simulink model "Copy_of_AB_Final_of_MPC_Bandwidth_Result"  (R2022b)
settings: Solver=FixedStepDiscrete  StartTime=0.0  StopTime=Inf  FixedStep=100e-6  RelTol=1e-3  EnableMultiTasking=on
undefined symbols (not defined in the file): C28x, CPU1, CPU2, CurrentBypassValue, DiscIntNeverNeededParam, Down, GPTRIP1SEL, TZ1, Up
libraries: c2802xlib x31, simulink x22, dspstat3 x17, dspsigops x9, c2837xDlib x6, c280xlib x5, PID_Lib x2, c2000lib x1, spsAlphaBetaZerotoabcLib x1, spsAlphaBetaZerotodq0Lib x1
(part 3 of 8)

== system Copy_of_AB_Final_of_MPC_Bandwidth_Result/Subsystem1/Subsystem ==
  PWM1 : Inport
  PWM2 : Inport  Port=2
  PWM3 : Inport  Port=3
  Trip : Inport  Port=4
  Constant12 : Constant  Value=uint32(4999)
  Constant13 : Constant  Value=uint32(0)
  Constant16 : Constant  Value=uint32(4999)
  Constant17 : Constant  Value=uint32(0)
  Constant6 : Constant  Value=uint32(4999)
  Constant7 : Constant  Value=uint32(0)
  Data Type Conversion18 : DataTypeConversion  OutDataTypeStr=uint32  SaturateOnIntegerOverflow=off  RndMeth=Floor
  Data Type Conversion19 : DataTypeConversion  OutDataTypeStr=uint32  SaturateOnIntegerOverflow=off  RndMeth=Floor
  Data Type Conversion5 : DataTypeConversion  OutDataTypeStr=uint32  SaturateOnIntegerOverflow=off  RndMeth=Floor
  From : From
  From1 : From
  From2 : From
  Gain : Gain
  Goto : Goto
  Saturation Dynamic1 : simulink/Discontinuities/Saturation Dynamic  OutMin=[]  OutMax=[]  OutDataTypeStr=Inherit: Same as second input  OutDataType=fixdt(1, 16)  OutScaling=2^-10  DoSatur=off
  Saturation Dynamic2 : simulink/Discontinuities/Saturation Dynamic  OutMin=[]  OutMax=[]  OutDataTypeStr=Inherit: Same as second input  OutDataType=fixdt(1, 16)  OutScaling=2^-10  DoSatur=off
  Saturation Dynamic3 : simulink/Discontinuities/Saturation Dynamic  OutMin=[]  OutMax=[]  OutDataTypeStr=Inherit: Same as second input  OutDataType=fixdt(1, 16)  OutScaling=2^-10  DoSatur=off
  ePWM5 : c2802xlib/ePWM  PwmType=C2000_Type4  useModule=ePWM1  ePWMxLINKTBPRD=Not Linked  periodUnits=Clock cycles  timerSource=Specify via dialog  timerPeriod_clk=5000  timerPeriod_sec=0.0001  tbshadow=Counter equals to zero  countingMode=Up-Down  phaseActiveEnable=Disable  phaseDirection=Count down after sync  phaseActive=0  synchronizationEnable=off  dcaevt1Sync=off  dcbevt1Sync=off  synchronizationOption=Disable  dcbevt1SyncOut=off  dcaevt1SyncOut=off  cmpdSyncOut=off  cmpcSyncOut=off  cmpbSyncOut=off  zeroSyncOut=off  swfSyncOut=off  perSynchronizationOption=Counter equals to period (CTR=PRD)  clockPrescale=1  HSclockPrescale=1  enswap=off  ePWMxAStatus=on  ePWMxAactionLogic1=Do nothing  ePWMxAactionLogic2=Do nothing  ePWMxAactionLogic3=Clear  ePWMxAactionLogic4=Set  ePWMxAactionLogic5=Do nothing  ePWMxAactionLogic6=Do nothing  ePWMxACSFenable=off  ePWMxACSFvalue=Forcing disable  ePWMxASFreload=Zero  ePWMxBStatus=off  ePWMxBactionLogic1=Set  ePWMxBactionLogic2=Clear  ePWMxBactionLogic3=Do nothing  ePWMxBactionLogic4=Do nothing  ePWMxBactionLogic5=Clear  ePWMxBactionLogic6=Set  ePWMxBCSFenable=off  ePWMxBCSFvalue=Forcing disable  ePWMxBSFreload=Zero  ePWNxBOutWay=off  ePWMxLINKCMPA=Not Linked  CMPAUnits=Clock cycles  CMPASource=Input port  CMPAValue_per=50  CMPAValue_clk=0  enCMPAshadow=Counter equals to zero (CTR=Zero)  ePWMxLINKCMPB=Not Linked  CMPBUnits=Clock cycles  CMPBSource=Specify via dialog  CMPBValue_per=50  CMPBValue_clk=0  enCMPBshadow=Counter equals to zero (CTR=Zero)  ePWMxLINKCMPC=Not Linked  CMPCUnits=Clock cycles  CMPCSource=Specify via dialog  CMPCValue_per=50  CMPCValue_clk=0  enCMPCshadow=Counter equals to zero (CTR=Zero)  ePWMxLINKCMPD=Not Linked  CMPDUnits=Clock cycles  CMPDSource=Specify via dialog  CMPDValue_per=50  CMPDValue_clk=32000  enCMPDshadow=Counter equals to zero (CTR=Zero)  enableDBePWMxA=on  enableDBePWMxB=on  enhalfcycle=off  DBpolarity=Active high complementary (AHC)  DBedgeDelay=Positive  DBSource_ePWMxA=ePWMxA  DBSource_ePWMxB=ePWMxA  DBPeriodUnits=Seconds  DBperiodSource=Specify via dialog  REDperiod=250  FEDperiod=250  REDperiod_sec=500e-9  FEDperiod_sec=500e-9  LoadModeDBRED=Immediate without using shadow  LoadModeDBFED=Immediate without using shadow  adcstartModuleA=on  adcrequestEventA=First event  adcstartEventA=Digital Compare Module A Event 1 start of conversion (DCAEVT1.soc)  adcstartEventA_type2=Counter equals to period (CTR=PRD)  adcstartModuleB=off  adcrequestEventB=First event  adcstartEventB=Counter equals to zero (CTR=Zero)  adcstartEventB_type2=Counter equals to zero (CTR=Zero)  intEn=off  intPrd=First event  intSel=Counter equals to zero (CTR=Zero)  intSel_type2=Counter equals to zero (CTR=Zero)  hrpe=off  enHRPWM=off  HRPWM_LoadMode=Counter equals to period (CTR=PRD)  HRPWM_CTLMode=Duty or Period control mode  HRPWM_EDGMode=Both edge  hrpeb=off  enHRPWMB=off  HRPWM_LoadModeB=Counter equals to zero (CTR=ZERO)  HRPWM_CTLModeB=Duty or Period control mode  HRPWM_EDGModeB=Both edge  enHRDBRED=off  enHRDBFED=off  enSFO=on  enautoconv=on  chopperEnable=off  chopperFrequency=1  chopperFirstwidth=1  chopperDuty=12.5%  tripZonesource=Input port  tzselOSHT1=off  tzselOSHT2=off  tzselOSHT3=off  tzselOSHDCAEV1=off  tzselOSHDCBEV1=off  tzselCBC1=off  tzselCBC2=off  tzselCBC3=off  tzselCBCDCAEV2=off  tzselCBCDCBEV2=off  tzselOSHT4=off  tzselOSHT5=off  tzselOSHT6=off  tzselCBC4=off  tzselCBC5=off  tzselCBC6=off  enTzOstIntr=off  enTzCbcIntr=off  enTzDCAEVT1Intr=off  enTzDCAEVT2Intr=off  enTzDCBEVT1Intr=off  enTzDCBEVT2Intr=off  ePWMxAforced=Low  ePWMxBforced=Low  DCAEVT1forced=No action  DCBEVT1forced=No action  DCAEVT2forced=No action  DCBEVT2forced=No action  dcah=Trip Zone 1 input (TZ1)  dcal=Trip Zone 2 input (TZ2)  dcbh=Trip Zone 1 input (TZ1)  dcbl=Trip Zone 2 input (TZ2)  dcah_type2=GPTRIP1SEL/(TZ1)  dcal_type2=GPTRIP1SEL/(TZ1)  dcbh_type2=GPTRIP1SEL/(TZ1)  dcbl_type2=GPTRIP1SEL/(TZ1)  gendcaevt1=Event disabled  gendcaevt2=Event disabled  gendcbevt1=Event disabled  gendcbevt2=Event disabled  dcaevt1src=DCAEVT1 with sync  dcaevt2src=DCAEVT2 with sync  dcbevt1src=DCBEVT1 with sync  dcbevt2src=DCBEVT2 with sync  pulsesel=Counter equals to zero (CTR=Zero)  blankinv=off  blankoffset=0  blankwidth=0  evsrcsel=Filtered version of DCAEVT1 (DCAEVT1FILT)  encape=off
  ePWM6 : c2802xlib/ePWM  PwmType=C2000_Type4  useModule=ePWM2  ePWMxLINKTBPRD=Not Linked  periodUnits=Clock cycles  timerSource=Specify via dialog  timerPeriod_clk=5000  timerPeriod_sec=0.0001  tbshadow=Counter equals to zero  countingMode=Up-Down  phaseActiveEnable=Disable  phaseDirection=Count down after sync  phaseActive=0  synchronizationEnable=off  dcaevt1Sync=off  dcbevt1Sync=off  synchronizationOption=Disable  dcbevt1SyncOut=off  dcaevt1SyncOut=off  cmpdSyncOut=off  cmpcSyncOut=off  cmpbSyncOut=off  zeroSyncOut=off  swfSyncOut=off  perSynchronizationOption=Counter equals to period (CTR=PRD)  clockPrescale=1  HSclockPrescale=1  enswap=off  ePWMxAStatus=on  ePWMxAactionLogic1=Do nothing  ePWMxAactionLogic2=Do nothing  ePWMxAactionLogic3=Clear  ePWMxAactionLogic4=Set  ePWMxAactionLogic5=Do nothing  ePWMxAactionLogic6=Do nothing  ePWMxACSFenable=off  ePWMxACSFvalue=Forcing disable  ePWMxASFreload=Zero  ePWMxBStatus=off  ePWMxBactionLogic1=Set  ePWMxBactionLogic2=Clear  ePWMxBactionLogic3=Do nothing  ePWMxBactionLogic4=Do nothing  ePWMxBactionLogic5=Clear  ePWMxBactionLogic6=Set  ePWMxBCSFenable=off  ePWMxBCSFvalue=Forcing disable  ePWMxBSFreload=Zero  ePWNxBOutWay=off  ePWMxLINKCMPA=Not Linked  CMPAUnits=Clock cycles  CMPASource=Input port  CMPAValue_per=50  CMPAValue_clk=0  enCMPAshadow=Counter equals to zero (CTR=Zero)  ePWMxLINKCMPB=Not Linked  CMPBUnits=Clock cycles  CMPBSource=Specify via dialog  CMPBValue_per=50  CMPBValue_clk=0  enCMPBshadow=Counter equals to zero (CTR=Zero)  ePWMxLINKCMPC=Not Linked  CMPCUnits=Clock cycles  CMPCSource=Specify via dialog  CMPCValue_per=50  CMPCValue_clk=0  enCMPCshadow=Counter equals to zero (CTR=Zero)  ePWMxLINKCMPD=Not Linked  CMPDUnits=Clock cycles  CMPDSource=Specify via dialog  CMPDValue_per=50  CMPDValue_clk=32000  enCMPDshadow=Counter equals to zero (CTR=Zero)  enableDBePWMxA=on  enableDBePWMxB=on  enhalfcycle=off  DBpolarity=Active high complementary (AHC)  DBedgeDelay=Positive  DBSource_ePWMxA=ePWMxA  DBSource_ePWMxB=ePWMxA  DBPeriodUnits=Seconds  DBperiodSource=Specify via dialog  REDperiod=250  FEDperiod=250  REDperiod_sec=500e-9  FEDperiod_sec=500e-9  LoadModeDBRED=Immediate without using shadow  LoadModeDBFED=Immediate without using shadow  adcstartModuleA=off  adcrequestEventA=First event  adcstartEventA=Digital Compare Module A Event 1 start of conversion (DCAEVT1.soc)  adcstartEventA_type2=Counter equals to zero (CTR=Zero)  adcstartModuleB=off  adcrequestEventB=First event  adcstartEventB=Counter equals to zero (CTR=Zero)  adcstartEventB_type2=Counter equals to zero (CTR=Zero)  intEn=off  intPrd=First event  intSel=Counter equals to zero (CTR=Zero)  intSel_type2=Counter equals to zero (CTR=Zero)  hrpe=off  enHRPWM=off  HRPWM_LoadMode=Counter equals to period (CTR=PRD)  HRPWM_CTLMode=Duty or Period control mode  HRPWM_EDGMode=Both edge  hrpeb=off  enHRPWMB=off  HRPWM_LoadModeB=Counter equals to zero (CTR=ZERO)  HRPWM_CTLModeB=Duty or Period control mode  HRPWM_EDGModeB=Both edge  enHRDBRED=off  enHRDBFED=off  enSFO=on  enautoconv=on  chopperEnable=off  chopperFrequency=1  chopperFirstwidth=1  chopperDuty=12.5%  tripZonesource=Input port  tzselOSHT1=off  tzselOSHT2=off  tzselOSHT3=off  tzselOSHDCAEV1=off  tzselOSHDCBEV1=off  tzselCBC1=off  tzselCBC2=off  tzselCBC3=off  tzselCBCDCAEV2=off  tzselCBCDCBEV2=off  tzselOSHT4=off  tzselOSHT5=off  tzselOSHT6=off  tzselCBC4=off  tzselCBC5=off  tzselCBC6=off  enTzOstIntr=off  enTzCbcIntr=off  enTzDCAEVT1Intr=off  enTzDCAEVT2Intr=off  enTzDCBEVT1Intr=off  enTzDCBEVT2Intr=off  ePWMxAforced=Low  ePWMxBforced=Low  DCAEVT1forced=No action  DCBEVT1forced=No action  DCAEVT2forced=No action  DCBEVT2forced=No action  dcah=Trip Zone 1 input (TZ1)  dcal=Trip Zone 2 input (TZ2)  dcbh=Trip Zone 1 input (TZ1)  dcbl=Trip Zone 2 input (TZ2)  dcah_type2=GPTRIP1SEL/(TZ1)  dcal_type2=GPTRIP1SEL/(TZ1)  dcbh_type2=GPTRIP1SEL/(TZ1)  dcbl_type2=GPTRIP1SEL/(TZ1)  gendcaevt1=Event disabled  gendcaevt2=Event disabled  gendcbevt1=Event disabled  gendcbevt2=Event disabled  dcaevt1src=DCAEVT1 with sync  dcaevt2src=DCAEVT2 with sync  dcbevt1src=DCBEVT1 with sync  dcbevt2src=DCBEVT2 with sync  pulsesel=Counter equals to zero (CTR=Zero)  blankinv=off  blankoffset=0  blankwidth=0  evsrcsel=Filtered version of DCAEVT1 (DCAEVT1FILT)  encape=off
  ePWM7 : c2802xlib/ePWM  PwmType=C2000_Type4  useModule=ePWM3  ePWMxLINKTBPRD=Not Linked  periodUnits=Clock cycles  timerSource=Specify via dialog  timerPeriod_clk=5000  timerPeriod_sec=0.0001  tbshadow=Counter equals to zero  countingMode=Up-Down  phaseActiveEnable=Disable  phaseDirection=Count down after sync  phaseActive=0  synchronizationEnable=off  dcaevt1Sync=off  dcbevt1Sync=off  synchronizationOption=Disable  dcbevt1SyncOut=off  dcaevt1SyncOut=off  cmpdSyncOut=off  cmpcSyncOut=off  cmpbSyncOut=off  zeroSyncOut=off  swfSyncOut=off  perSynchronizationOption=Counter equals to period (CTR=PRD)  clockPrescale=1  HSclockPrescale=1  enswap=off  ePWMxAStatus=on  ePWMxAactionLogic1=Do nothing  ePWMxAactionLogic2=Do nothing  ePWMxAactionLogic3=Clear  ePWMxAactionLogic4=Set  ePWMxAactionLogic5=Do nothing  ePWMxAactionLogic6=Do nothing  ePWMxACSFenable=off  ePWMxACSFvalue=Forcing disable  ePWMxASFreload=Zero  ePWMxBStatus=off  ePWMxBactionLogic1=Set  ePWMxBactionLogic2=Clear  ePWMxBactionLogic3=Do nothing  ePWMxBactionLogic4=Do nothing  ePWMxBactionLogic5=Clear  ePWMxBactionLogic6=Set  ePWMxBCSFenable=off  ePWMxBCSFvalue=Forcing disable  ePWMxBSFreload=Zero  ePWNxBOutWay=off  ePWMxLINKCMPA=Not Linked  CMPAUnits=Clock cycles  CMPASource=Input port  CMPAValue_per=50  CMPAValue_clk=0  enCMPAshadow=Counter equals to zero (CTR=Zero)  ePWMxLINKCMPB=Not Linked  CMPBUnits=Clock cycles  CMPBSource=Specify via dialog  CMPBValue_per=50  CMPBValue_clk=0  enCMPBshadow=Counter equals to zero (CTR=Zero)  ePWMxLINKCMPC=Not Linked  CMPCUnits=Clock cycles  CMPCSource=Specify via dialog  CMPCValue_per=50  CMPCValue_clk=0  enCMPCshadow=Counter equals to zero (CTR=Zero)  ePWMxLINKCMPD=Not Linked  CMPDUnits=Clock cycles  CMPDSource=Specify via dialog  CMPDValue_per=50  CMPDValue_clk=32000  enCMPDshadow=Counter equals to zero (CTR=Zero)  enableDBePWMxA=on  enableDBePWMxB=on  enhalfcycle=off  DBpolarity=Active high complementary (AHC)  DBedgeDelay=Positive  DBSource_ePWMxA=ePWMxA  DBSource_ePWMxB=ePWMxA  DBPeriodUnits=Seconds  DBperiodSource=Specify via dialog  REDperiod=250  FEDperiod=250  REDperiod_sec=500e-9  FEDperiod_sec=500e-9  LoadModeDBRED=Immediate without using shadow  LoadModeDBFED=Immediate without using shadow  adcstartModuleA=off  adcrequestEventA=First event  adcstartEventA=Digital Compare Module A Event 1 start of conversion (DCAEVT1.soc)  adcstartEventA_type2=Counter equals to zero (CTR=Zero)  adcstartModuleB=off  adcrequestEventB=First event  adcstartEventB=Counter equals to zero (CTR=Zero)  adcstartEventB_type2=Counter equals to zero (CTR=Zero)  intEn=off  intPrd=First event  intSel=Counter equals to zero (CTR=Zero)  intSel_type2=Counter equals to zero (CTR=Zero)  hrpe=off  enHRPWM=off  HRPWM_LoadMode=Counter equals to period (CTR=PRD)  HRPWM_CTLMode=Duty or Period control mode  HRPWM_EDGMode=Both edge  hrpeb=off  enHRPWMB=off  HRPWM_LoadModeB=Counter equals to zero (CTR=ZERO)  HRPWM_CTLModeB=Duty or Period control mode  HRPWM_EDGModeB=Both edge  enHRDBRED=off  enHRDBFED=off  enSFO=on  enautoconv=on  chopperEnable=off  chopperFrequency=1  chopperFirstwidth=1  chopperDuty=12.5%  tripZonesource=Input port  tzselOSHT1=off  tzselOSHT2=off  tzselOSHT3=off  tzselOSHDCAEV1=off  tzselOSHDCBEV1=off  tzselCBC1=off  tzselCBC2=off  tzselCBC3=off  tzselCBCDCAEV2=off  tzselCBCDCBEV2=off  tzselOSHT4=off  tzselOSHT5=off  tzselOSHT6=off  tzselCBC4=off  tzselCBC5=off  tzselCBC6=off  enTzOstIntr=off  enTzCbcIntr=off  enTzDCAEVT1Intr=off  enTzDCAEVT2Intr=off  enTzDCBEVT1Intr=off  enTzDCBEVT2Intr=off  ePWMxAforced=Low  ePWMxBforced=Low  DCAEVT1forced=No action  DCBEVT1forced=No action  DCAEVT2forced=No action  DCBEVT2forced=No action  dcah=Trip Zone 1 input (TZ1)  dcal=Trip Zone 2 input (TZ2)  dcbh=Trip Zone 1 input (TZ1)  dcbl=Trip Zone 2 input (TZ2)  dcah_type2=GPTRIP1SEL/(TZ1)  dcal_type2=GPTRIP1SEL/(TZ1)  dcbh_type2=GPTRIP1SEL/(TZ1)  dcbl_type2=GPTRIP1SEL/(TZ1)  gendcaevt1=Event disabled  gendcaevt2=Event disabled  gendcbevt1=Event disabled  gendcbevt2=Event disabled  dcaevt1src=DCAEVT1 with sync  dcaevt2src=DCAEVT2 with sync  dcbevt1src=DCBEVT1 with sync  dcbevt2src=DCBEVT2 with sync  pulsesel=Counter equals to zero (CTR=Zero)  blankinv=off  blankoffset=0  blankwidth=0  evsrcsel=Filtered version of DCAEVT1 (DCAEVT1FILT)  encape=off
  wires:
  Data Type Conversion5/1 -> ePWM5/1
  Constant13/1 -> Saturation Dynamic3/3
  Constant6/1 -> Saturation Dynamic1/1
  Constant12/1 -> Saturation Dynamic3/1
  Constant7/1 -> Saturation Dynamic1/3
  Saturation Dynamic1/1 -> Data Type Conversion5/1
  Constant16/1 -> Saturation Dynamic2/1
  Data Type Conversion18/1 -> ePWM6/1
  Data Type Conversion19/1 -> ePWM7/1
  Saturation Dynamic3/1 -> Data Type Conversion19/1
  Constant17/1 -> Saturation Dynamic2/3
  Saturation Dynamic2/1 -> Data Type Conversion18/1
  PWM1/1 -> Saturation Dynamic1/2
  PWM3/1 -> Saturation Dynamic3/2
  PWM2/1 -> Saturation Dynamic2/2
  From/1 -> ePWM5/2
  From1/1 -> ePWM6/2
  From2/1 -> ePWM7/2
  Trip/1 -> Gain/1
  Gain/1 -> Goto/1

== system Copy_of_AB_Final_of_MPC_Bandwidth_Result/Subsystem1/Subsystem1 ==
  In1 : Inport
  In2 : Inport  Port=2
  Enable : EnablePort  StatesWhenEnabling=reset
  Add : Sum
  Add3 : Sum
  Bus Creator : BusCreator  Inputs=2
  Bus Selector1 : BusSelector  OutputSignals=signal1,signal2
  CodeGeneration : Subsystem  TreatAsAtomicUnit=on
  Constant3 : Constant  Value=100  OutDataTypeStr=single
  Counter Limited : simulink/Sources/Counter Limited  uplimit=599  tsamp=-1
  Data : Subsystem  TreatAsAtomicUnit=on
  Data_Conditioning : Subsystem
  End : Subsystem  TreatAsAtomicUnit=on
  Gain6 : Gain  Gain=1000  OutDataTypeStr=single
  Gain7 : Gain  Gain=1000  OutDataTypeStr=single
  If : If  IfExpression=u1 == 0  ElseIfExpressions=u1 == 599
  Merge : Merge  Inputs=3
  Merge1 : Merge  Inputs=3
  Mux : Mux  Inputs=2
  Mux1 : Mux  Inputs=2
  Start : Subsystem  TreatAsAtomicUnit=on
  Width : Width  OutDataTypeMode=All ports same datatype  DataType=uint16
  wires:
  Start/2(Iteration) -> Merge1/1
  Constant3/1 -> Add/2, Add3/1
  Counter Limited/1 -> If/1
  Data_Conditioning/1(Out1) -> Width/1, Start/1(Data), End/1(Data), Data/1(Data)
  End/1(Data_out) -> Merge/2
  End/2(Iteration) -> Merge1/2
  If/3 -> Data/Action
  Add/1 -> Gain6/1
  Data/2(Iteration) -> Merge1/3
  Merge1/1 -> Mux/2  "SCI_Tx_Iteration"
  Bus Selector1/1 -> Add/1  "<signal1>"
  Start/1(Data_out) -> Merge/1
  Add3/1 -> Gain7/1
  Mux1/1 -> Data_Conditioning/1(In1)
  In1/1 -> Bus Creator/1
  Merge/1 -> Mux/1  "SCI_Tx_Data"
  If/2 -> End/Action
  Data/1(Data_out) -> Merge/3
  Bus Creator/1 -> Bus Selector1/1
  Width/1 -> Start/2(Data_width), Data/2(Data_width), End/2(Data_width)
  Mux/1 -> CodeGeneration/1(Input)
  In2/1 -> Bus Creator/2
  Gain7/1 -> Mux1/2
  Bus Selector1/2 -> Add3/2  "<signal2>"
  If/1 -> Start/Action
  Gain6/1 -> Mux1/1

== system Copy_of_AB_Final_of_MPC_Bandwidth_Result/Subsystem1/Subsystem2 ==
  In1 : Inport
  In2 : Inport  Port=2
  Enable : EnablePort  StatesWhenEnabling=reset
  Add : Sum
  Add3 : Sum
  Bus Creator : BusCreator  Inputs=2
  Bus Selector1 : BusSelector  OutputSignals=signal1,signal2
  CodeGeneration : Subsystem  TreatAsAtomicUnit=on
  Constant3 : Constant  Value=10  OutDataTypeStr=single
  Counter Limited : simulink/Sources/Counter Limited  uplimit=599  tsamp=-1
  Data : Subsystem  TreatAsAtomicUnit=on
  Data_Conditioning : Subsystem
  End : Subsystem  TreatAsAtomicUnit=on
  Gain6 : Gain  Gain=1000  OutDataTypeStr=single
  Gain7 : Gain  Gain=1000  OutDataTypeStr=single
  If : If  IfExpression=u1 == 0  ElseIfExpressions=u1 == 599
  Merge : Merge  Inputs=3
  Merge1 : Merge  Inputs=3
  Mux : Mux  Inputs=2
  Mux1 : Mux  Inputs=2
  Start : Subsystem  TreatAsAtomicUnit=on
  Width : Width  OutDataTypeMode=All ports same datatype  DataType=uint16
  wires:
  Start/2(Iteration) -> Merge1/1
  Constant3/1 -> Add/2, Add3/1
  Counter Limited/1 -> If/1
  Data_Conditioning/1(Out1) -> Width/1, Start/1(Data), End/1(Data), Data/1(Data)
  End/1(Data_out) -> Merge/2
  End/2(Iteration) -> Merge1/2
  If/3 -> Data/Action
  Add/1 -> Gain6/1
  Data/2(Iteration) -> Merge1/3
  Merge1/1 -> Mux/2  "SCI_Tx_Iteration"
  Bus Selector1/1 -> Add/1  "<signal1>"
  Start/1(Data_out) -> Merge/1
  Add3/1 -> Gain7/1
  Mux1/1 -> Data_Conditioning/1(In1)
  In1/1 -> Bus Creator/1
  Merge/1 -> Mux/1  "SCI_Tx_Data"
  If/2 -> End/Action
  Data/1(Data_out) -> Merge/3
  Bus Creator/1 -> Bus Selector1/1
  Width/1 -> Start/2(Data_width), Data/2(Data_width), End/2(Data_width)
  Mux/1 -> CodeGeneration/1(Input)
  In2/1 -> Bus Creator/2
  Gain7/1 -> Mux1/2
  Bus Selector1/2 -> Add3/2  "<signal2>"
  If/1 -> Start/Action
  Gain6/1 -> Mux1/1

== system Copy_of_AB_Final_of_MPC_Bandwidth_Result/Subsystem1/Subsystem6 ==
  In1 : Inport
  In2 : Inport  Port=2
  theta : Inport  Port=3
  Add : Sum
  Add1 : Sum  Inputs=-+
  Cos : Trigonometry  Operator=cos
  Cos1 : Trigonometry
  From : From
  From4 : From
  Goto : Goto
  Product{,1..3} (4 alike) : Product
  Id : Outport
  Iq : Outport  Port=2
  wires:
  theta/1 -> Cos1/1, Cos/1
  In1/1 -> Goto/1
  In2/1 -> [b]
  From/1 -> Product/1
  Cos/1 -> [cosine]
  Cos1/1 -> [sinee]
  [cosine] -> Product/2
  [b] -> Product1/1
  [sinee] -> Product1/2
  Product/1 -> Add/1
  Product1/1 -> Add/2
  Add/1 -> Id/1
  [sinee] -> Product2/2
  [b] -> Product3/1
  Product3/1 -> Add1/2
  From4/1 -> Product2/1
  Product2/1 -> Add1/1
  [cosine] -> Product3/2
  Add1/1 -> Iq/1

== system Copy_of_AB_Final_of_MPC_Bandwidth_Result/Subsystem1/System Outputs ==

== system Copy_of_AB_Final_of_MPC_Bandwidth_Result/Subsystem1/VoltageReferenceCalculation ==
  MPCC_f32RGrid : Inport
  MPCC_f32LGrid : Inport  Port=2
  MPCC_f32SamplingPeriod : Inport  Port=3
  MPCC_f32AngularFrequency : Inport  Port=4
  MPCC_f32DGridCurrent : Inport  Port=5
  MPCC_f32QGridCurrent : Inport  Port=6
  MPCC_f32HarmonicDGridCurrent : Inport  Port=7
  MPCC_f32HarmonicQGridCurrent : Inport  Port=8
  MPCC_f32DGridVoltage : Inport  Port=9
  MPCC_f32QGridVoltage : Inport  Port=10
  MPCC_f32DGridCurrentReference : Inport  Port=11
  MPCC_f32HarmonicDGridCurrentReference : Inport  Port=12
  MPCC_f32QGridCurrentReference : Inport  Port=13
  MPCC_f32HarmonicQGridCurrentReference : Inport  Port=14
  MPCC_f32ElectricalAngle : Inport  Port=15
  MPCC_f32DCLinkVoltage : Inport  Port=16
  MPCC_f32HarmonicDGridVoltage : Inport  Port=17
  MPCC_f32HarmonicQGridVoltage : Inport  Port=18
  ElectricalAngleCompensation : Subsystem
  PredictiveTermsCalculation : Subsystem
  VdqVoltageReferenceCalculation : Subsystem
  MPCC_f32DVoltageReference : Outport
  MPCC_f32QVoltageReference : Outport  Port=2
  MPCC_f32ElectricalAngle_K_1 : Outport  Port=3
  MPCC_f32Predictionterm_A : Outport  Port=4
  MPCC_f32Predictionterm_B : Outport  Port=5
  MPCC_f32Predictionterm_C : Outport  Port=6
  wires:
  MPCC_f32RGrid/1 -> PredictiveTermsCalculation/1(MPCC_f32RGrid)
  PredictiveTermsCalculation/1(MPCC_f32Predictionterm_A) -> MPCC_f32Predictionterm_A/1, [MPCC_f32Predictionterm_A]
  PredictiveTermsCalculation/3(MPCC_f32Predictionterm_C) -> [MPCC_f32Predictionterm_C], MPCC_f32Predictionterm_C/1
  [MPCC_f32Predictionterm_A] -> VdqVoltageReferenceCalculation/1(MPCC_f32Predictionterm_A)
  [MPCC_f32Predictionterm_B] -> VdqVoltageReferenceCalculation/2(MPCC_f32Predictionterm_B)
  [MPCC_f32Predictionterm_C] -> VdqVoltageReferenceCalculation/3(MPCC_f32Predictionterm_C)
  MPCC_f32QGridCurrentReference/1 -> VdqVoltageReferenceCalculation/12(MPCC_f32QGridCurrentReference)
  MPCC_f32QGridCurrent/1 -> VdqVoltageReferenceCalculation/5(MPCC_f32QGridCurrent)
  [MPCC_f32SamplingPeriod] -> VdqVoltageReferenceCalculation/15(MPCC_f32SamplingPeriod)
  MPCC_f32DGridCurrent/1 -> VdqVoltageReferenceCalculation/4(MPCC_f32DGridCurrent)
  MPCC_f32HarmonicDGridCurrent/1 -> VdqVoltageReferenceCalculation/6(MPCC_f32HarmonicDGridCurrent)
  MPCC_f32HarmonicDGridCurrentReference/1 -> VdqVoltageReferenceCalculation/11(MPCC_f32HarmonicDGridCurrentReference)
  MPCC_f32HarmonicQGridCurrent/1 -> VdqVoltageReferenceCalculation/7(MPCC_f32HarmonicQGridCurrent)
  MPCC_f32HarmonicQGridCurrentReference/1 -> VdqVoltageReferenceCalculation/13(MPCC_f32HarmonicQGridCurrentReference)
  [MPCC_f32LGrid] -> VdqVoltageReferenceCalculation/14(MPCC_f32LGrid)
  MPCC_f32DGridCurrentReference/1 -> VdqVoltageReferenceCalculation/10(MPCC_f32DGridCurrentReference)
  MPCC_f32QGridVoltage/1 -> VdqVoltageReferenceCalculation/9(MPCC_f32QGridVoltage)
  MPCC_f32DGridVoltage/1 -> VdqVoltageReferenceCalculation/8(MPCC_f32DGridVoltage)
  MPCC_f32LGrid/1 -> [MPCC_f32LGrid]
  MPCC_f32SamplingPeriod/1 -> [MPCC_f32SamplingPeriod]
  [MPCC_f32LGrid] -> PredictiveTermsCalculation/2(MPCC_f32LGrid)
  [MPCC_f32SamplingPeriod] -> PredictiveTermsCalculation/3(MPCC_f32SamplingPeriod)
  VdqVoltageReferenceCalculation/1(MPCC_f32DVoltageReference) -> MPCC_f32DVoltageReference/1
  VdqVoltageReferenceCalculation/2(MPCC_f32QVoltageReference) -> MPCC_f32QVoltageReference/1
  [MPCC_f32SamplingPeriod] -> ElectricalAngleCompensation/1(MPCC_f32SamplingPeriod)
  MPCC_f32ElectricalAngle/1 -> [MPCC_f32ElectricalAngle]
  MPCC_f32AngularFrequency/1 -> [MPCC_f32AngularFrequency]
  [MPCC_f32AngularFrequency] -> ElectricalAngleCompensation/2(MPCC_f32AngularFrequency)
  [MPCC_f32ElectricalAngle] -> ElectricalAngleCompensation/3(MPCC_f32ElectricalAngle)
  ElectricalAngleCompensation/1(MPCC_f32ElectricalAngle_K_1) -> MPCC_f32ElectricalAngle_K_1/1
  [MPCC_f32AngularFrequency] -> PredictiveTermsCalculation/4(MPCC_f32AngularFrequency)
  PredictiveTermsCalculation/2(MPCC_f32Predictionterm_B) -> MPCC_f32Predictionterm_B/1, [MPCC_f32Predictionterm_B]
  MPCC_f32DCLinkVoltage/1 -> VdqVoltageReferenceCalculation/16(MPCC_f32DCLinkVoltage)
  MPCC_f32HarmonicDGridVoltage/1 -> VdqVoltageReferenceCalculation/17(MPCC_f32HarmonicDGridVoltage)
  MPCC_f32HarmonicQGridVoltage/1 -> VdqVoltageReferenceCalculation/18(MPCC_f32HarmonicQGridVoltage)

== system Copy_of_AB_Final_of_MPC_Bandwidth_Result/Subsystem1/dq_abc1 ==
  theta : Inport
  vd : Inport  Port=2
  vq : Inport  Port=3
  Cast To Single : DataTypeConversion  OutDataTypeStr=single  SaturateOnIntegerOverflow=off  RndMeth=Floor
  Cast To Single1 : DataTypeConversion  OutDataTypeStr=single  SaturateOnIntegerOverflow=off  RndMeth=Floor
  Cast To Single2 : DataTypeConversion  OutDataTypeStr=single  SaturateOnIntegerOverflow=off  RndMeth=Floor
  Subsystem6 : Subsystem
  Ia : Outport
  Ib : Outport  Port=2
  Ic : Outport  Port=3
  wires:
  theta/1 -> Subsystem6/3(theta)
  vq/1 -> Subsystem6/2(In2)
  vd/1 -> Subsystem6/1(In1)
  Subsystem6/3(Ic) -> Cast To Single2/1
  Subsystem6/2(Ib) -> Cast To Single1/1
  Subsystem6/1(Ia) -> Cast To Single/1
  Cast To Single/1 -> Ia/1
  Cast To Single1/1 -> Ib/1
  Cast To Single2/1 -> Ic/1

== system Copy_of_AB_Final_of_MPC_Bandwidth_Result/Subsystem3/LPF ==
  u_k : Inport
  Add : Sum  Inputs=+-
  Add1 : Sum
  Delay : Delay  DelayLength=1
  Gain : Gain  Gain=single(100/1100)
  y_k : Outport
  wires:
  Delay/1 -> Add/2, Add1/2
  Add/1 -> Gain/1
  Gain/1 -> Add1/1
  Add1/1 -> y_k/1, Delay/1
  u_k/1 -> Add/1

== system Copy_of_AB_Final_of_MPC_Bandwidth_Result/Subsystem3/LPF1 ==
  u_k : Inport
  Add : Sum  Inputs=+-
  Add1 : Sum
  Delay : Delay  DelayLength=1
  Gain : Gain  Gain=single(100/1100)
  y_k : Outport
  wires:
  Delay/1 -> Add/2, Add1/2
  Add/1 -> Gain/1
  Gain/1 -> Add1/1
  Add1/1 -> y_k/1, Delay/1
  u_k/1 -> Add/1

== system Copy_of_AB_Final_of_MPC_Bandwidth_Result/Subsystem3/LPF2 ==
  u_k : Inport
  Add : Sum  Inputs=+-
  Add1 : Sum
  Delay : Delay  DelayLength=1
  Gain : Gain  Gain=single(100/1100)
  y_k : Outport
  wires:
  Delay/1 -> Add/2, Add1/2
  Add/1 -> Gain/1
  Gain/1 -> Add1/1
  Add1/1 -> y_k/1, Delay/1
  u_k/1 -> Add/1

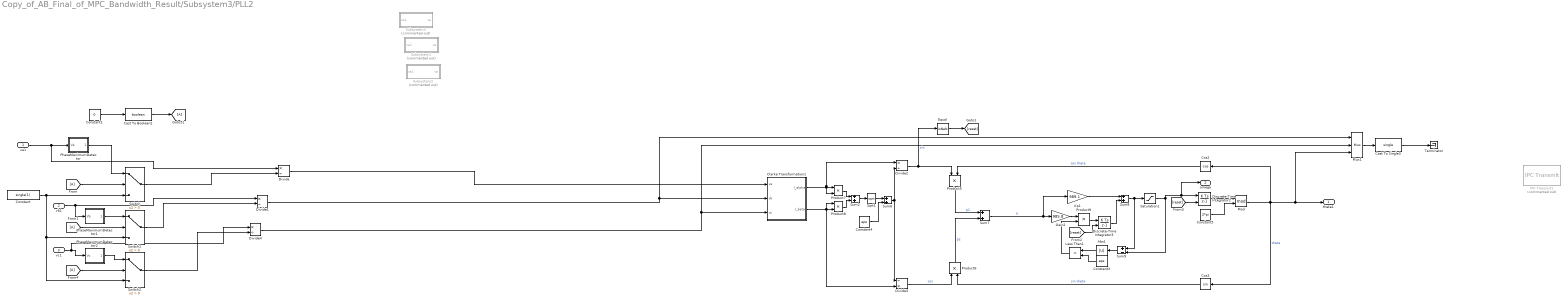
== system Copy_of_AB_Final_of_MPC_Bandwidth_Result/Subsystem3/PLL2 ==
  va1 : Inport
  vb1 : Inport  Port=2
  vc1 : Inport  Port=3
  Abs1 : Abs  SaturateOnIntegerOverflow=off
  Cast To Boolean2 : DataTypeConversion  OutDataTypeStr=boolean  SaturateOnIntegerOverflow=off  RndMeth=Floor
  Cast To Single3 : DataTypeConversion  OutDataTypeStr=single  SaturateOnIntegerOverflow=off  RndMeth=Floor
  Clarke Transformation1 : Subsystem
  Constant : Constant  Value=single(1)
  Constant1 : Constant  Value=0
  Constant3 : Constant  Value=eps  OutDataTypeStr=single  SampleTime=-1
  Constant4 : Constant  Value=eps  OutDataTypeStr=single
  Constant5 : Constant  Value=2*pi  OutDataTypeStr=single  SampleTime=-1
  Cos2 : Trigonometry  Operator=cos
  Cos3 : Trigonometry
  Discrete-Time Integrator2 : DiscreteIntegrator  ExternalReset=either  SampleTime=-1  ICPrevOutput=DiscIntNeverNeededParam  ICPrevScaledInput=DiscIntNeverNeededParam
  Discrete-Time Integrator3 : DiscreteIntegrator  ExternalReset=either  SampleTime=-1  ICPrevOutput=DiscIntNeverNeededParam  ICPrevScaledInput=DiscIntNeverNeededParam
  Divide : Product  Inputs=*/  RndMeth=Zero  SaturateOnIntegerOverflow=on
  Divide1 : Product  Inputs=*/  RndMeth=Zero  SaturateOnIntegerOverflow=on
  Divide2 : Product  Inputs=*/
  Divide3 : Product  Inputs=/*
  Divide4 : Product  Inputs=*/  RndMeth=Zero  SaturateOnIntegerOverflow=on
  Equal : RelationalOperator  Operator=isNaN  OutDataTypeStr=boolean  RndMeth=Simplest  InputSameDT=off
  From : From
  From1 : From
  From4 : From
  Gain2 : Gain  Gain=985.8  SaturateOnIntegerOverflow=on  OutDataTypeStr=Inherit: Same as input  ParamDataTypeStr=Inherit: Same as input
  Goto51 : Goto
  IPC Transmit1 : c2837xDlib/IPC Transmit  Commented=on  blkParamProc=F2837x  SelectDestination=C28x (CPU1/CPU2)  SelectChannel=0  EnableBlocking=off
  Kp1 : Gain  Gain=989.1  SaturateOnIntegerOverflow=on  OutDataTypeStr=Inherit: Same as input  ParamDataTypeStr=Inherit: Same as input
  Less Than1 : RelationalOperator  Operator=<  OutDataTypeStr=boolean  RndMeth=Simplest  InputSameDT=off
  Mod : Math  Operator=mod
  Mux1 : Mux  Inputs=3
  PhaseMaximumDetector : Subsystem
  PhaseMaximumDetector1 : Subsystem
  PhaseMaximumDetector2 : Subsystem
  Product{5..9} (5 alike) : Product
  Saturation1 : Saturate  UpperLimit=inf  LowerLimit=-inf
  Sqrt1 : Sqrt  OutDataTypeStr=single  IntermediateResultsDataTypeStr=single
  Subsystem1 : Subsystem  Commented=on
  Subsystem2 : Subsystem  Commented=on
  Subsystem3 : Subsystem  Commented=on
  Sum2 : Sum
  Sum6 : Sum  OutDataTypeStr=single
  Sum7 : Sum
  Sum8 : Sum
  Sum9 : Sum  Inputs=+-
  Switch : Switch  Criteria=u2 > Threshold  SaturateOnIntegerOverflow=off  InputSameDT=off
  Switch1 : Switch  Criteria=u2 > Threshold  SaturateOnIntegerOverflow=off  InputSameDT=off
  Switch2 : Switch  Criteria=u2 > Threshold  SaturateOnIntegerOverflow=off  InputSameDT=off
  Terminator : Terminator
  theta1 : Outport
  omega : Outport  Port=2
  wires:
  Clarke Transformation1/1(I_alpha) -> Divide2/1, Product7/1, Product7/2
  Saturation1/1 -> Sum9/2, omega/1, Discrete-Time Integrator2/1
  Product9/1 -> Discrete-Time Integrator3/1
  Sum9/1 -> Abs1/1
  Abs1/1 -> Less Than1/1
  Cos3/1 -> Product6/2  "sin theta"
  Product7/1 -> Sum2/1
  [reset] -> Discrete-Time Integrator2/2
  Discrete-Time Integrator3/1 -> Sum8/2
  Product8/1 -> Sum2/2
  Divide2/1 -> Product5/1, Equal/1  "sin"
  Product6/1 -> Sum7/2  "p2"
  Sum8/1 -> Sum9/1, Saturation1/1
  Mod/1 -> Cos2/1, Mux1/3, theta1/1, Cos3/1  "theta"
  Sum6/1 -> Divide3/1, Divide2/2
  Sum2/1 -> Sqrt1/1
  Divide3/1 -> Product6/1  "cos"
  Clarke Transformation1/2(I_beta) -> Product8/2, Product8/1, Divide3/2
  Cos2/1 -> Product5/2  "cos theta"
  Constant5/1 -> Mod/2
  Product5/1 -> Sum7/1  "p1"
  Sum7/1 -> Kp1/1, Gain2/1  "e"
  Equal/1 -> [reset]
  Kp1/1 -> Sum8/1
  Constant3/1 -> Less Than1/2
  Less Than1/1 -> Product9/2
  [reset] -> Discrete-Time Integrator3/2
  Sqrt1/1 -> Sum6/1
  Gain2/1 -> Product9/1
  Discrete-Time Integrator2/1 -> Mod/1
  Constant4/1 -> Sum6/2
  Divide/1 -> Clarke Transformation1/1(va)
  Divide1/1 -> Mux1/1, Clarke Transformation1/2(vb)
  Divide4/1 -> Mux1/2, Clarke Transformation1/3(vc)
  Mux1/1 -> Cast To Single3/1
  va1/1 -> Divide/1, PhaseMaximumDetector/1(Va)
  PhaseMaximumDetector/1(Vamax) -> Switch/1
  Switch2/1 -> Divide4/2
  Switch1/1 -> Divide1/2
  PhaseMaximumDetector1/1(Vbmax) -> Switch1/1
  vb1/1 -> Divide1/1, PhaseMaximumDetector1/1(Vb)
  Constant1/1 -> Cast To Boolean2/1
  Switch/1 -> Divide/2
  From1/1 -> Switch1/2
  vc1/1 -> Divide4/1, PhaseMaximumDetector2/1(Vc)
  Constant/1 -> Switch2/3, Switch1/3, Switch/3
  From4/1 -> Switch2/2
  PhaseMaximumDetector2/1(Vcmax) -> Switch2/1
  From/1 -> Switch/2
  Cast To Boolean2/1 -> Goto51/1
  ? -> IPC Transmit1/1
  Cast To Single3/1 -> Terminator/1

== system Copy_of_AB_Final_of_MPC_Bandwidth_Result/Subsystem3/PLL_Loop1 ==
  MPCC_f32GridVoltageA : Inport
  MPCC_f32GridVoltageB : Inport  Port=2
  MPCC_f32GridVoltageC : Inport  Port=3
  ABCtoAlphaBeta : Subsystem
  Add : Sum  Inputs=+-  OutDataTypeStr=Inherit: Inherit via back propagation
  Add1 : Sum  Inputs=+-
  Add2 : Sum
  Add3 : Sum
  Add4 : Sum
  Amplitude : Fcn  Expr=sqrt(u(1)^2+u(2)^2)
  Cast To Single : DataTypeConversion  OutDataTypeStr=single  SaturateOnIntegerOverflow=off  RndMeth=Floor
  Cast To Single1 : DataTypeConversion  OutDataTypeStr=single  SaturateOnIntegerOverflow=off  RndMeth=Floor
  Constant : Constant  Value=single(2*2*pi*500*1/sqrt(2))  VectorParams1D=off
  Constant1 : Constant  Value=single(500*500*4*pi*pi)
  Constant2 : Constant  Value=inf
  Constant3 : Constant  Value=boolean(1)
  Constant4 : Constant  Value=boolean(0)
  Constant5 : Constant  Value=single(2*pi*50)
  Constant6 : Constant  Value=single(2*2*pi*30*(1/sqrt(2)))
  Constant7 : Constant  Value=single(0)
  Constant8 : Constant  Value=-inf
  Constant9 : Constant  Value=single(30*30*4*pi*pi)
  Discrete integrator 2π wrapping1 : Subsystem
  Gain : Gain  Gain=0.5
  Gain1 : Gain  Gain=0.5
  LPF : DiscreteFilter  Numerator=[0 (2*pi*14*100e-6)]  Denominator=[1 (2*pi*14*100e-6-1)]  InitialStates=50/14/100e-6
  Mux : Mux  Inputs=2
  Mux1 : Mux  Inputs=3
  Normalization : Fcn  Expr=u(3)/(u(1)+(1e-6)*(u(1)==0))
  PI : PID_Lib/PI  SystemSampleTime=-1  VariantActivationTime=update diagram  Latency=0  AutoFrameSizeCalculation=off
  SOGI 1st : Subsystem
  SOGI 1st2 : Subsystem  Commented=on
  SOGI 1st3 : Subsystem
  SOGI 1st4 : Subsystem  Commented=on
  Scope1 : Scope  NumInputPorts=2
  Subsystem6 : Subsystem
  Terminator : Terminator
  Terminator2 : Terminator
  Terminator3 : Terminator
  ω1 : Constant  Value=single(2*pi*50)  OutDataTypeStr=single
  ω2 : Constant  Value=single(2*pi*50)  OutDataTypeStr=single
  MPCC_f32AngularFrequency : Outport
  MPCC_f32ElectricalAngle : Outport  Port=2
  wires:
  Constant7/1 -> Add/1
  Constant2/1 -> PI/4
  Constant3/1 -> PI/6
  Constant4/1 -> PI/7
  PI/2 -> Terminator/1
  PI/4 -> Terminator2/1
  PI/5 -> Terminator3/1
  MPCC_f32GridVoltageB/1 -> [MPCC_f32GridVoltageB]
  MPCC_f32GridVoltageC/1 -> [MPCC_f32GridVoltageC]
  Constant8/1 -> PI/5
  PI/1 -> Cast To Single/1
  [MPCC_f32GridVoltageA] -> ABCtoAlphaBeta/1(In1)
  [MPCC_f32GridVoltageB] -> ABCtoAlphaBeta/2(In2)
  [MPCC_f32GridVoltageC] -> ABCtoAlphaBeta/3(In3)
  Add1/1 -> Gain/1
  Add2/1 -> Gain1/1
  Gain/1 -> Subsystem6/1(In1)
  Gain1/1 -> Subsystem6/2(In2)
  Constant5/1 -> PI/8
  Subsystem6/1(Id) -> Mux1/2, Mux/1
  Subsystem6/2(Iq) -> Mux1/3, Mux/2
  Mux/1 -> Amplitude/1
  Mux1/1 -> Normalization/1
  Amplitude/1 -> Mux1/1
  Cast To Single/1 -> Add3/2
  ω2/1 -> Add3/1
  Add3/1 -> Discrete integrator 2π wrapping1/1(ω)
  Discrete integrator 2π wrapping1/1(θ) -> Scope1/2, [MPCC_f32ElectricalAngle], MPCC_f32ElectricalAngle/1
  PI/3 -> Cast To Single1/1
  ω1/1 -> Add4/1
  Cast To Single1/1 -> Add4/2
  [MPCC_f32ElectricalAngle] -> Subsystem6/3(theta)
  Add4/1 -> LPF/1
  [MPCC_f32AngularFrequency] -> SOGI 1st/1(w)
  [MPCC_f32AngularFrequency] -> SOGI 1st3/1(w)
  MPCC_f32GridVoltageA/1 -> Scope1/1, [MPCC_f32GridVoltageA]
  Normalization/1 -> PI/1
  Constant/1 -> PI/2
  Constant1/1 -> PI/3
  LPF/1 -> [MPCC_f32AngularFrequency], MPCC_f32AngularFrequency/1
  ABCtoAlphaBeta/1(Out1) -> SOGI 1st/2(Vαβ)
  ABCtoAlphaBeta/2(Vαβ) -> SOGI 1st3/2(Vαβ)
  SOGI 1st/1(v) -> Add1/1
  SOGI 1st/2(qv) -> Add2/2
  SOGI 1st3/2(qv) -> Add1/2
  SOGI 1st3/1(v) -> Add2/1

== system Copy_of_AB_Final_of_MPC_Bandwidth_Result/Subsystem3/RateLimiter ==
  Up : Inport
  Ts : Inport  Port=2
  Lo : Inport  Port=3
  U : Inport  Port=4
  Xo : Inport  Port=5
  Rs : Inport  Port=6
  Add1 : Sum  Inputs=+-
  Add2 : Sum
  Data Type Duplicate : DataTypeDuplicate  NumInputPorts=7
  Delay : Delay  DelayLength=1  InitialConditionSource=Input port  ExternalReset=Rising
      settings: InputPortMap=u0,r5,p4
  Product : Product
  Product1 : Product
  Saturation Dynamic : simulink/Discontinuities/Saturation Dynamic  OutMin=[]  OutMax=[]  OutDataTypeStr=Inherit: Same as second input  OutDataType=fixdt(1, 16)  OutScaling=2^-10  DoSatur=off
  Y : Outport
  wires:
  Xo/1 -> Delay/3
  Product1/1 -> Data Type Duplicate/3, Saturation Dynamic/3
  Add1/1 -> Data Type Duplicate/4, Saturation Dynamic/2
  Add2/1 -> Data Type Duplicate/1, Y/1, Delay/1
  Delay/1 -> Data Type Duplicate/2, Add1/2, Add2/2
  U/1 -> Data Type Duplicate/5, Add1/1
  Saturation Dynamic/1 -> Data Type Duplicate/7, Add2/1
  Product/1 -> Data Type Duplicate/6, Saturation Dynamic/1
  Rs/1 -> Delay/2
  Ts/1 -> Product1/1, Product/2
  Lo/1 -> Product1/2
  Up/1 -> Product/1

== system Copy_of_AB_Final_of_MPC_Bandwidth_Result/Subsystem3/RateLimiter1 ==
  Up : Inport
  Ts : Inport  Port=2
  Lo : Inport  Port=3
  U : Inport  Port=4
  Xo : Inport  Port=5
  Rs : Inport  Port=6
  Add1 : Sum  Inputs=+-
  Add2 : Sum
  Data Type Duplicate : DataTypeDuplicate  NumInputPorts=7
  Delay : Delay  DelayLength=1  InitialConditionSource=Input port  ExternalReset=Rising
      settings: InputPortMap=u0,r5,p4
  Product : Product
  Product1 : Product
  Saturation Dynamic : simulink/Discontinuities/Saturation Dynamic  OutMin=[]  OutMax=[]  OutDataTypeStr=Inherit: Same as second input  OutDataType=fixdt(1, 16)  OutScaling=2^-10  DoSatur=off
  Y : Outport
  wires:
  Xo/1 -> Delay/3
  Product1/1 -> Data Type Duplicate/3, Saturation Dynamic/3
  Add1/1 -> Data Type Duplicate/4, Saturation Dynamic/2
  Add2/1 -> Data Type Duplicate/1, Y/1, Delay/1
  Delay/1 -> Data Type Duplicate/2, Add1/2, Add2/2
  U/1 -> Data Type Duplicate/5, Add1/1
  Saturation Dynamic/1 -> Data Type Duplicate/7, Add2/1
  Product/1 -> Data Type Duplicate/6, Saturation Dynamic/1
  Rs/1 -> Delay/2
  Ts/1 -> Product1/1, Product/2
  Lo/1 -> Product1/2
  Up/1 -> Product/1

== system Copy_of_AB_Final_of_MPC_Bandwidth_Result/Subsystem3/RateLimiter2 ==
  Up : Inport
  Ts : Inport  Port=2
  Lo : Inport  Port=3
  U : Inport  Port=4
  Xo : Inport  Port=5
  Rs : Inport  Port=6
  Add1 : Sum  Inputs=+-
  Add2 : Sum
  Data Type Duplicate : DataTypeDuplicate  NumInputPorts=7
  Delay : Delay  DelayLength=1  InitialConditionSource=Input port  ExternalReset=Rising
      settings: InputPortMap=u0,r5,p4
  Product : Product
  Product1 : Product
  Saturation Dynamic : simulink/Discontinuities/Saturation Dynamic  OutMin=[]  OutMax=[]  OutDataTypeStr=Inherit: Same as second input  OutDataType=fixdt(1, 16)  OutScaling=2^-10  DoSatur=off
  Y : Outport
  wires:
  Xo/1 -> Delay/3
  Product1/1 -> Data Type Duplicate/3, Saturation Dynamic/3
  Add1/1 -> Data Type Duplicate/4, Saturation Dynamic/2
  Add2/1 -> Data Type Duplicate/1, Y/1, Delay/1
  Delay/1 -> Data Type Duplicate/2, Add1/2, Add2/2
  U/1 -> Data Type Duplicate/5, Add1/1
  Saturation Dynamic/1 -> Data Type Duplicate/7, Add2/1
  Product/1 -> Data Type Duplicate/6, Saturation Dynamic/1
  Rs/1 -> Delay/2
  Ts/1 -> Product1/1, Product/2
  Lo/1 -> Product1/2
  Up/1 -> Product/1

== system Copy_of_AB_Final_of_MPC_Bandwidth_Result/Subsystem5/Subsystem3 ==
  DiffInput : Inport
  Trigger : Inport  Port=2
  Cast1 : DataTypeConversion  OutDataTypeStr=int8  SaturateOnIntegerOverflow=off  RndMeth=Floor
  Mean1 : dspstat3/Mean  run=on  InputProcessing=Columns as channels (frame based)  reset_popup=Rising edge  directionMode=Each column  dimension=1  roiEnable=off  roiType=Rectangles  roiPortion=Entire ROI  roiOutput=Individual statistics for each ROI  roiFlag=off  roundingMode=Floor  overflowMode=off  outputDataTypeStr=Inherit: Same as accumulator  outputMin=[]  outputMax=[]  outputLastDataTypeStr=Inherit: Same as accumulator
  Mean : Outport
  wires:
  Cast1/1 -> Mean1/2
  DiffInput/1 -> Mean1/1
  Mean1/1 -> Mean/1
  Trigger/1 -> Cast1/1

== system Copy_of_AB_Final_of_MPC_Bandwidth_Result/Subsystem5/Subsystem4 ==
  DiffInput : Inport
  Trigger : Inport  Port=2
  Cast1 : DataTypeConversion  OutDataTypeStr=int8  SaturateOnIntegerOverflow=off  RndMeth=Floor
  Mean1 : dspstat3/Mean  run=on  InputProcessing=Columns as channels (frame based)  reset_popup=Rising edge  directionMode=Each column  dimension=1  roiEnable=off  roiType=Rectangles  roiPortion=Entire ROI  roiOutput=Individual statistics for each ROI  roiFlag=off  roundingMode=Floor  overflowMode=off  outputDataTypeStr=Inherit: Same as accumulator  outputMin=[]  outputMax=[]  outputLastDataTypeStr=Inherit: Same as accumulator
  Mean : Outport
  wires:
  Cast1/1 -> Mean1/2
  DiffInput/1 -> Mean1/1
  Mean1/1 -> Mean/1
  Trigger/1 -> Cast1/1

== system Copy_of_AB_Final_of_MPC_Bandwidth_Result/Subsystem5/Subsystem6 ==
  DiffInput : Inport
  Trigger : Inport  Port=2
  Cast1 : DataTypeConversion  OutDataTypeStr=int8  SaturateOnIntegerOverflow=off  RndMeth=Floor
  Mean1 : dspstat3/Mean  run=on  InputProcessing=Columns as channels (frame based)  reset_popup=Rising edge  directionMode=Each column  dimension=1  roiEnable=off  roiType=Rectangles  roiPortion=Entire ROI  roiOutput=Individual statistics for each ROI  roiFlag=off  roundingMode=Floor  overflowMode=off  outputDataTypeStr=Inherit: Same as accumulator  outputMin=[]  outputMax=[]  outputLastDataTypeStr=Inherit: Same as accumulator
  Mean : Outport
  wires:
  Cast1/1 -> Mean1/2
  DiffInput/1 -> Mean1/1
  Mean1/1 -> Mean/1
  Trigger/1 -> Cast1/1

== system Copy_of_AB_Final_of_MPC_Bandwidth_Result/Voltage_Loop/Subsystem5 ==
  MPCC_f32DCLink : Inport
  Cast To Single1 : DataTypeConversion  OutDataTypeStr=single  SaturateOnIntegerOverflow=off  RndMeth=Floor
  LPF : Subsystem
  MPCC_f32DCLinkFiltered : Outport
  wires:
  LPF/1(y_k) -> Cast To Single1/1
  MPCC_f32DCLink/1 -> LPF/1(u_k)
  Cast To Single1/1 -> MPCC_f32DCLinkFiltered/1  "Iau"

== system Copy_of_AB_Final_of_MPC_Bandwidth_Result/Subsystem1/ABCtoDQO/ABCtoDQOCurrent ==
  PI_f32GridCurrentA : Inport
  PI_f32GridCurrentB : Inport  Port=2
  PI_f32GridCurrentC : Inport  Port=3
  PI_f32ElectricalAngle : Inport  Port=4
  ABCtoO : Subsystem
  ABCtoQ : Subsystem
  ABCtoQ1 : Subsystem
  PI_f32DGridCurrent : Outport
  PI_f32QGridCurrent : Outport  Port=2
  PI_f32OGridCurrent : Outport  Port=3
  wires:
  ABCtoQ/1(PI_f32QGridCurrent) -> PI_f32QGridCurrent/1
  [PI_f32GridCurrentC] -> ABCtoQ/3(PI_f32GridCurrentC)
  PI_f32GridCurrentC/1 -> [PI_f32GridCurrentC]
  PI_f32GridCurrentA/1 -> [PI_f32GridCurrentA]
  [PI_f32GridCurrentB] -> ABCtoO/2(PI_f32GridCurrentB)
  [PI_f32GridCurrentA] -> ABCtoO/1(PI_f32GridCurrentA)
  [PI_f32ElectricalAngle] -> ABCtoQ/4(PI_f32ElectricalAngle)
  [PI_f32GridCurrentA] -> ABCtoQ/1(PI_f32GridCurrentA)
  [PI_f32GridCurrentC] -> ABCtoO/3(PI_f32GridCurrentC)
  [PI_f32GridCurrentB] -> ABCtoQ/2(PI_f32GridCurrentB)
  PI_f32ElectricalAngle/1 -> [PI_f32ElectricalAngle]
  PI_f32GridCurrentB/1 -> [PI_f32GridCurrentB]
  ABCtoQ1/1(MPCC_f32QGridVoltage) -> PI_f32DGridCurrent/1
  ABCtoO/1(PI_f32OGridCurrent) -> PI_f32OGridCurrent/1
  [PI_f32GridCurrentA] -> ABCtoQ1/1(MPCC_f32GridVoltageA)
  [PI_f32GridCurrentB] -> ABCtoQ1/2(MPCC_f32GridVoltageB)
  [PI_f32GridCurrentC] -> ABCtoQ1/3(MPCC_f32GridVoltageC)
  [PI_f32ElectricalAngle] -> ABCtoQ1/4(MPCC_f32ElectricalAngle)

== system Copy_of_AB_Final_of_MPC_Bandwidth_Result/Subsystem1/ABCtoDQO/ABCtoDQOVoltage ==
  PI_f32GridCurrentA : Inport
  PI_f32GridCurrentB : Inport  Port=2
  PI_f32GridCurrentC : Inport  Port=3
  PI_f32ElectricalAngle : Inport  Port=4
  ABCtoO : Subsystem
  ABCtoQ : Subsystem
  ABCtoQ1 : Subsystem
  PI_f32DGridCurrent : Outport
  PI_f32QGridCurrent : Outport  Port=2
  PI_f32OGridCurrent : Outport  Port=3
  wires:
  ABCtoQ/1(PI_f32QGridCurrent) -> PI_f32QGridCurrent/1
  [PI_f32GridCurrentC] -> ABCtoQ/3(PI_f32GridCurrentC)
  PI_f32GridCurrentC/1 -> [PI_f32GridCurrentC]
  PI_f32GridCurrentA/1 -> [PI_f32GridCurrentA]
  [PI_f32GridCurrentB] -> ABCtoO/2(PI_f32GridCurrentB)
  [PI_f32GridCurrentA] -> ABCtoO/1(PI_f32GridCurrentA)
  [PI_f32ElectricalAngle] -> ABCtoQ/4(PI_f32ElectricalAngle)
  [PI_f32GridCurrentA] -> ABCtoQ/1(PI_f32GridCurrentA)
  [PI_f32GridCurrentC] -> ABCtoO/3(PI_f32GridCurrentC)
  [PI_f32GridCurrentB] -> ABCtoQ/2(PI_f32GridCurrentB)
  PI_f32ElectricalAngle/1 -> [PI_f32ElectricalAngle]
  PI_f32GridCurrentB/1 -> [PI_f32GridCurrentB]
  ABCtoQ1/1(MPCC_f32QGridVoltage) -> PI_f32DGridCurrent/1
  ABCtoO/1(PI_f32OGridCurrent) -> PI_f32OGridCurrent/1
  [PI_f32GridCurrentA] -> ABCtoQ1/1(MPCC_f32GridVoltageA)
  [PI_f32GridCurrentB] -> ABCtoQ1/2(MPCC_f32GridVoltageB)
  [PI_f32GridCurrentC] -> ABCtoQ1/3(MPCC_f32GridVoltageC)
  [PI_f32ElectricalAngle] -> ABCtoQ1/4(MPCC_f32ElectricalAngle)

== system Copy_of_AB_Final_of_MPC_Bandwidth_Result/Subsystem1/ABCtoDQO/abc_dq ==
  theta : Inport
  a : Inport  Port=2
  b : Inport  Port=3
  c : Inport  Port=4
  Subsystem5 : Subsystem
  Subsystem6 : Subsystem
  Id : Outport
  Iq : Outport  Port=2
  wires:
  c/1 -> Subsystem5/3(In3)
  Subsystem5/2(Iq) -> Iq/1, Subsystem6/2(In2)
  b/1 -> Subsystem5/2(In2)
  theta/1 -> Subsystem6/3(theta)
  Subsystem5/1(Id) -> Id/1, Subsystem6/1(In1)
  a/1 -> Subsystem5/1(In1)

== system Copy_of_AB_Final_of_MPC_Bandwidth_Result/Subsystem1/ABCtoDQO/abc_dq1 ==
  theta : Inport
  a : Inport  Port=2
  b : Inport  Port=3
  c : Inport  Port=4
  Subsystem5 : Subsystem
  Subsystem6 : Subsystem
  Id : Outport
  Iq : Outport  Port=2
  wires:
  c/1 -> Subsystem5/3(In3)
  Subsystem5/2(Iq) -> Iq/1, Subsystem6/2(In2)
  b/1 -> Subsystem5/2(In2)
  theta/1 -> Subsystem6/3(theta)
  Subsystem5/1(Id) -> Id/1, Subsystem6/1(In1)
  a/1 -> Subsystem5/1(In1)

== system Copy_of_AB_Final_of_MPC_Bandwidth_Result/Subsystem1/ABCtoDQO/abc_dq4 ==
  theta : Inport
  a : Inport  Port=2
  b : Inport  Port=3
  c : Inport  Port=4
  c1 : Inport  Port=5
  Add : Sum  Inputs=+-
  Add1 : Sum
  Product : Product
  Product1 : Product
  Scope : Scope
  Scope1 : Scope
  Subsystem5 : Subsystem
  Subsystem6 : Subsystem
  Id : Outport
  Iq : Outport  Port=2
  wires:
  c/1 -> Subsystem5/3(In3)
  b/1 -> Subsystem5/2(In2)
  Subsystem6/1(Id) -> Scope/1
  Subsystem6/2(Iq) -> Scope1/1
  a/1 -> Subsystem5/1(In1)
  Subsystem5/1(Out1) -> Product1/2, Add/1
  Subsystem5/2(Out2) -> Add1/2, Product/1
  theta/1 -> Product1/1, Product/2
  Product/1 -> Add/2
  Product1/1 -> Add1/1
  c1/1 -> Subsystem6/3(theta)
  Add/1 -> Id/1, Subsystem6/1(In1)
  Add1/1 -> Iq/1, Subsystem6/2(In2)

== system Copy_of_AB_Final_of_MPC_Bandwidth_Result/Subsystem1/AlphaBetaDutiesCalculation/AlphaBetaVoltageReferenceCalculation ==
  MPCC_f32DVoltageReference : Inport
  MPCC_f32QVoltageReference : Inport  Port=2
  MPCC_f32ElectricalAngle_K_1 : Inport  Port=3
  Add : Sum  Inputs=+-
  Add1 : Sum
  Product{,1..3} (4 alike) : Product
  Sin : Trigonometry  Operator=cos
  Sin1 : Trigonometry
  Sin2 : Trigonometry
  Sin3 : Trigonometry  Operator=cos
  MPCC_f32AlphaVoltageReference : Outport
  MPCC_f32BetaVoltageReference : Outport  Port=2
  wires:
  Sin2/1 -> Product2/1
  [MPCC_f32QVoltageReference] -> Product3/2
  Sin1/1 -> Product1/1
  Sin3/1 -> Product3/1
  Product/1 -> Add/1
  [MPCC_f32DVoltageReference] -> Product2/2
  [MPCC_f32ElectricalAngle_K_1] -> Sin2/1
  [MPCC_f32QVoltageReference] -> Product1/2
  Add1/1 -> MPCC_f32BetaVoltageReference/1
  Product2/1 -> Add1/1
  Product3/1 -> Add1/2
  [MPCC_f32ElectricalAngle_K_1] -> Sin3/1
  MPCC_f32DVoltageReference/1 -> [MPCC_f32DVoltageReference]
  Add/1 -> MPCC_f32AlphaVoltageReference/1
  [MPCC_f32ElectricalAngle_K_1] -> Sin/1
  [MPCC_f32DVoltageReference] -> Product/2
  MPCC_f32QVoltageReference/1 -> [MPCC_f32QVoltageReference]
  Product1/1 -> Add/2
  Sin/1 -> Product/1
  [MPCC_f32ElectricalAngle_K_1] -> Sin1/1
  MPCC_f32ElectricalAngle_K_1/1 -> [MPCC_f32ElectricalAngle_K_1]
